simulink model "model_reg_quality"  (R2024a)
settings: Solver=FixedStepAuto  StartTime=0.0  StopTime=4  FixedStep=0.00001  RelTol=1e-3
values from neighbouring files (symbols this model uses):
  A = [5 -5 -9 3; -5 5 -3 9; -9 -3 5 5; 3 9 5 5]    [obsreg.m]    (also in obsreg1.m; obsreg_k1.m; obsreg_k1_1.m; obsreg_k2.m)
  B = [2; 6; 6; 2]    [obsreg.m]    (also in obsreg1.m; obsreg_k1.m; obsreg_k1_1.m; obsreg_k2.m)
  K1 = -inv(R)*B'*P    [obsreg_k1.m]    (also in obsreg_k1_1.m; reg_quality1.m = -double(inv(R + B'*P*B) * B'*P*(A - beta*eye(3))))
  K2 = -inv(R)*B'*P    [obsreg_k2.m]    (also in obsreg_k2_1.m; reg_quality2.m = -double(inv(R + B'*P*B) * B'*P*(A - beta*eye(3))))
  K3 = Y / P    [obsreg_k3.m]    (also in obsreg_k3_1.m = -inv(R)*B'*P; reg_quality3.m = -double(inv(R + B'*P*B) * B'*P*(A - beta*eye(3))))
  K4 = -double(inv(R + B'*P*B) * B'*P*(A - beta*eye(3)))    [reg_quality4.m]
settings Model: Creator=ventus  LastModifiedBy=ventus

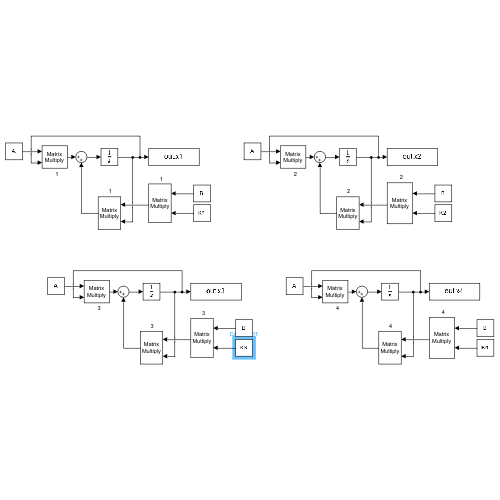
[thumbnail: Simulink's stored preview of the top-level diagram]
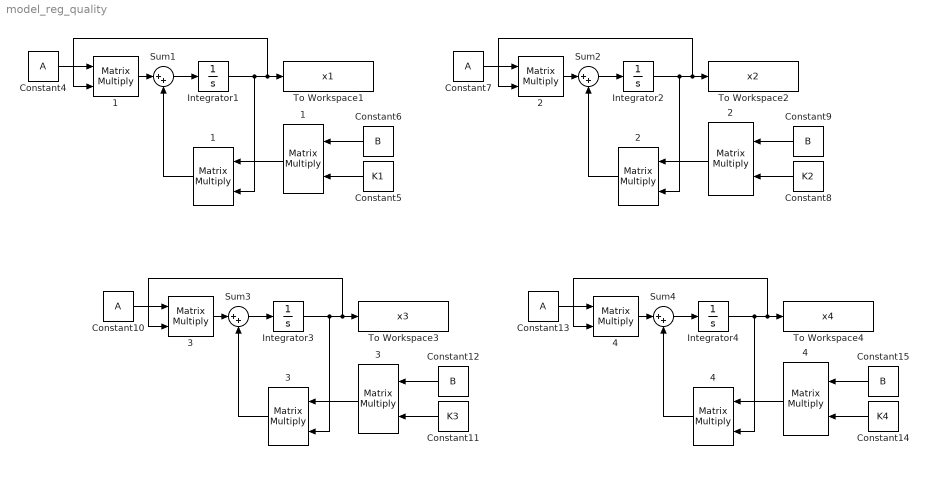
== system model_reg_quality ==
     {1..4} (4 alike) : Product  Multiplication=Matrix(*)
    {1..4} (4 alike) : Product  Multiplication=Matrix(*)
   {1..4} (4 alike) : Product  Multiplication=Matrix(*)
  Constant{4,7,10,13} (4 alike) : Constant  Value=A  VectorParams1D=off
  Constant11 : Constant  Value=K3  VectorParams1D=off
  Constant{6,9,12,15} (4 alike) : Constant  Value=B  VectorParams1D=off
  Constant14 : Constant  Value=K4  VectorParams1D=off
  Constant5 : Constant  Value=K1  VectorParams1D=off
  Constant8 : Constant  Value=K2  VectorParams1D=off
  Integrator{1..4} (4 alike) : Integrator  InitialCondition=[1; 1; 1]
  Sum{1..4} (4 alike) : Sum  Inputs=|++
  To Workspace1 : ToWorkspace  VariableName=x1  SaveFormat=Timeseries  SampleTime=-1
  To Workspace2 : ToWorkspace  VariableName=x2  SaveFormat=Timeseries  SampleTime=-1
  To Workspace3 : ToWorkspace  VariableName=x3  SaveFormat=Timeseries  SampleTime=-1
  To Workspace4 : ToWorkspace  VariableName=x4  SaveFormat=Timeseries  SampleTime=-1
  wires:
  Constant8/1 -> "  2"/2
  Constant14/1 -> "  4"/2
  Sum2/1 -> Integrator2/1
  Integrator2/1 -> To Workspace2/1, "   2"/2, " 2"/2
  Integrator3/1 -> To Workspace3/1, "   3"/2, " 3"/2
  "   2"/1 -> Sum2/1
  Constant6/1 -> "  1"/1
  Integrator4/1 -> To Workspace4/1, "   4"/2, " 4"/2
  "   4"/1 -> Sum4/1
  "  4"/1 -> " 4"/1
  " 3"/1 -> Sum3/2
  Constant9/1 -> "  2"/1
  Constant12/1 -> "  3"/1
  "   3"/1 -> Sum3/1
  " 4"/1 -> Sum4/2
  Constant15/1 -> "  4"/1
  "  2"/1 -> " 2"/1
  "  3"/1 -> " 3"/1
  Constant10/1 -> "   3"/1
  Sum1/1 -> Integrator1/1
  Constant7/1 -> "   2"/1
  Sum4/1 -> Integrator4/1
  Constant11/1 -> "  3"/2
  Sum3/1 -> Integrator3/1
  " 1"/1 -> Sum1/2
  Constant13/1 -> "   4"/1
  Constant5/1 -> "  1"/2
  "  1"/1 -> " 1"/1
  Constant4/1 -> "   1"/1
  " 2"/1 -> Sum2/2
  "   1"/1 -> Sum1/1
  Integrator1/1 -> To Workspace1/1, "   1"/2, " 1"/2
